simulink model "manipulator_cl"  (R2018b)
settings: Solver=ode45  StartTime=0.0  StopTime=4  RelTol=1e-6
values from neighbouring files (symbols this model uses):
  alpha_rel = 60*pi/180    (= 1.0471975512)    [parameters.m]
  kp1 = 160    [parameters.m]
  kp2 = 60    [parameters.m]
  kv1 = 11    [parameters.m]
  kv2 = 1.1    [parameters.m]
  rad_deg = 180/pi    (= 57.2957795131)    [parameters.m]
  sys_titop = directDynamicsSuper*tf(1, [1 0])    [titop_model.m]
undefined symbols (not defined in the file or in its folder): sys_phode
settings Model: Creator=a.brugnoli  LastModifiedBy=a.brugnoli

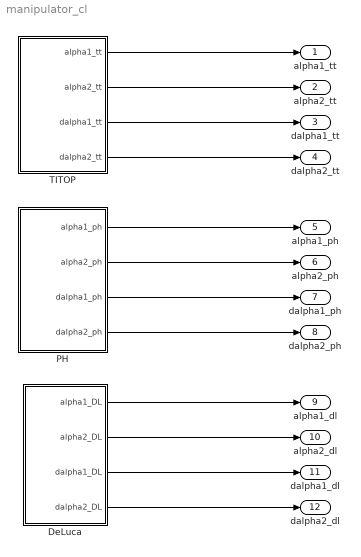
== system manipulator_cl ==
  DeLuca : Subsystem
  PH : Subsystem
  TITOP : Subsystem
  alpha1_tt : Outport
  alpha2_tt : Outport  Port=2
  dalpha1_tt : Outport  Port=3
  dalpha2_tt : Outport  Port=4
  alpha1_ph : Outport  Port=5
  alpha2_ph : Outport  Port=6
  dalpha1_ph : Outport  Port=7
  dalpha2_ph : Outport  Port=8
  alpha1_dl : Outport  Port=9
  alpha2_dl : Outport  Port=10
  dalpha1_dl : Outport  Port=11
  dalpha2_dl : Outport  Port=12
  wires:
  TITOP/1(alpha1_tt) -> alpha1_tt/1
  TITOP/2(alpha2_tt) -> alpha2_tt/1
  TITOP/3(dalpha1_tt) -> dalpha1_tt/1
  TITOP/4(dalpha2_tt) -> dalpha2_tt/1
  PH/1(alpha1_ph) -> alpha1_ph/1
  PH/2(alpha2_ph) -> alpha2_ph/1
  PH/3(dalpha1_ph) -> dalpha1_ph/1
  PH/4(dalpha2_ph) -> dalpha2_ph/1
  DeLuca/1(alpha1_DL) -> alpha1_dl/1
  DeLuca/2(alpha2_DL) -> alpha2_dl/1
  DeLuca/3(dalpha1_DL) -> dalpha1_dl/1
  DeLuca/4(dalpha2_DL) -> dalpha2_dl/1

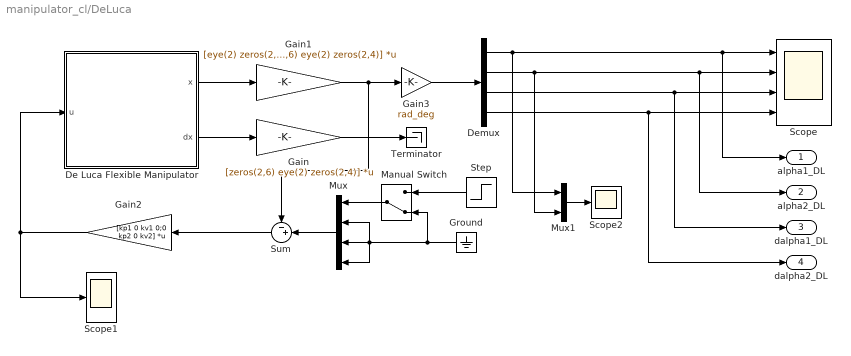
== system manipulator_cl/DeLuca ==
  De Luca Flexible Manipulator : Subsystem
  Demux : Demux
  Gain : Gain  Gain=[zeros(2,6) eye(2) zeros(2,4)]  Multiplication=Matrix(K*u) (u vector)
  Gain1 : Gain  Gain=[eye(2) zeros(2,10); zeros(2,6) eye(2) zeros(2,4)]  Multiplication=Matrix(K*u) (u vector)
  Gain2 : Gain  Gain="[kp1 0 kv1 0;0  kp2 0  kv2]"  Multiplication=Matrix(K*u) (u vector)
  Gain3 : Gain  Gain=rad_deg
  Ground : Ground
  Manual Switch : ManualSwitch  CurrentSetting=0
  Mux : Mux
  Mux1 : Mux  Inputs=2
  Scope : Scope  NumInputPorts=4
  Scope1 : Scope
  Scope2 : Scope
  Step : Step  After=alpha_rel  SampleTime=0
  Sum : Sum  Inputs=-+|
  Terminator : Terminator
  alpha1_DL : Outport
  alpha2_DL : Outport  Port=2
  dalpha1_DL : Outport  Port=3
  dalpha2_DL : Outport  Port=4
  wires:
  Gain/1 -> Terminator/1
  Mux1/1 -> Scope2/1
  Step/1 -> Manual Switch/1
  De Luca Flexible Manipulator/2(dx) -> Gain/1
  Mux/1 -> Sum/2
  Demux/1 -> alpha1_DL/1, Scope/1, Mux1/1
  Gain2/1 -> Scope1/1, De Luca Flexible Manipulator/1(u)
  Demux/2 -> alpha2_DL/1, Scope/2, Mux1/2
  Gain1/1 -> Gain3/1, Sum/1
  Demux/3 -> dalpha1_DL/1, Scope/3
  De Luca Flexible Manipulator/1(x) -> Gain1/1
  Gain3/1 -> Demux/1
  Ground/1 -> Manual Switch/2, Mux/2, Mux/4, Mux/3
  Demux/4 -> dalpha2_DL/1, Scope/4
  Sum/1 -> Gain2/1
  Manual Switch/1 -> Mux/1

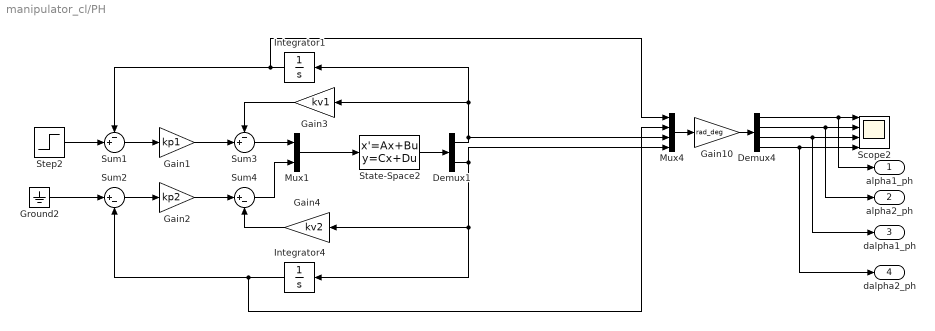
== system manipulator_cl/PH ==
  Demux1 : Demux  Outputs=2
  Demux4 : Demux
  Gain1 : Gain  Gain=kp1
  Gain10 : Gain  Gain=rad_deg
  Gain2 : Gain  Gain=kp2
  Gain3 : Gain  Gain=kv1
  Gain4 : Gain  Gain=kv2
  Ground2 : Ground
  Integrator1 : Integrator
  Integrator4 : Integrator
  Mux1 : Mux  Inputs=2
  Mux4 : Mux
  Scope2 : Scope  NumInputPorts=4
  State-Space2 : StateSpace  A=sys_phode.A  B=sys_phode.B  C=sys_phode.C  D=sys_phode.D  InitialCondition=0
  Step2 : Step  After=alpha_rel  SampleTime=0
  Sum1 : Sum  Inputs=-+|
  Sum2 : Sum  Inputs=|+-
  Sum3 : Sum  Inputs=-+|
  Sum4 : Sum  Inputs=|+-
  alpha1_ph : Outport
  alpha2_ph : Outport  Port=2
  dalpha1_ph : Outport  Port=3
  dalpha2_ph : Outport  Port=4
  wires:
  Gain1/1 -> Sum3/2
  Mux4/1 -> Gain10/1
  Gain3/1 -> Sum3/1
  Gain2/1 -> Sum4/1
  Demux4/1 -> alpha1_ph/1, Scope2/1
  Gain10/1 -> Demux4/1
  Sum2/1 -> Gain2/1
  Ground2/1 -> Sum2/1
  Sum1/1 -> Gain1/1
  Demux4/4 -> dalpha2_ph/1, Scope2/4
  Demux1/2 -> Integrator4/1, Gain4/1, Mux4/4
  Demux4/2 -> alpha2_ph/1, Scope2/2
  Integrator1/1 -> Mux4/1, Sum1/1
  Integrator4/1 -> Mux4/2, Sum2/2
  Step2/1 -> Sum1/2
  Demux1/1 -> Gain3/1, Integrator1/1, Mux4/3
  Mux1/1 -> State-Space2/1
  Demux4/3 -> dalpha1_ph/1, Scope2/3
  Sum4/1 -> Mux1/2
  Sum3/1 -> Mux1/1
  State-Space2/1 -> Demux1/1
  Gain4/1 -> Sum4/2

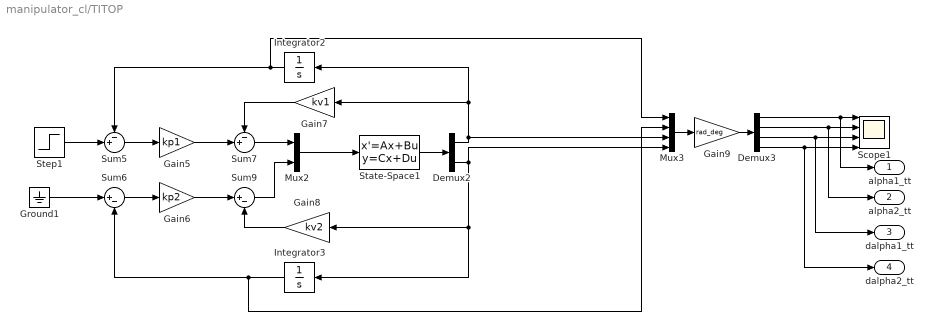
== system manipulator_cl/TITOP ==
  Demux2 : Demux  Outputs=2
  Demux3 : Demux
  Gain5 : Gain  Gain=kp1
  Gain6 : Gain  Gain=kp2
  Gain7 : Gain  Gain=kv1
  Gain8 : Gain  Gain=kv2
  Gain9 : Gain  Gain=rad_deg
  Ground1 : Ground
  Integrator2 : Integrator
  Integrator3 : Integrator
  Mux2 : Mux  Inputs=2
  Mux3 : Mux
  Scope1 : Scope  NumInputPorts=4
  State-Space1 : StateSpace  A=sys_titop.A  B=sys_titop.B  C=sys_titop.C  D=sys_titop.D  InitialCondition=0
  Step1 : Step  After=alpha_rel  SampleTime=0
  Sum5 : Sum  Inputs=-+|
  Sum6 : Sum  Inputs=|+-
  Sum7 : Sum  Inputs=-+|
  Sum9 : Sum  Inputs=|+-
  alpha1_tt : Outport
  alpha2_tt : Outport  Port=2
  dalpha1_tt : Outport  Port=3
  dalpha2_tt : Outport  Port=4
  wires:
  Gain5/1 -> Sum7/2
  Ground1/1 -> Sum6/1
  Gain7/1 -> Sum7/1
  State-Space1/1 -> Demux2/1
  Gain8/1 -> Sum9/2
  Demux3/3 -> dalpha1_tt/1, Scope1/3
  Demux2/1 -> Gain7/1, Integrator2/1, Mux3/3
  Integrator3/1 -> Mux3/2, Sum6/2
  Integrator2/1 -> Mux3/1, Sum5/1
  Sum9/1 -> Mux2/2
  Gain9/1 -> Demux3/1
  Demux2/2 -> Integrator3/1, Gain8/1, Mux3/4
  Demux3/4 -> dalpha2_tt/1, Scope1/4
  Mux3/1 -> Gain9/1
  Sum5/1 -> Gain5/1
  Sum7/1 -> Mux2/1
  Demux3/2 -> alpha2_tt/1, Scope1/2
  Mux2/1 -> State-Space1/1
  Sum6/1 -> Gain6/1
  Demux3/1 -> alpha1_tt/1, Scope1/1
  Gain6/1 -> Sum9/1
  Step1/1 -> Sum5/2

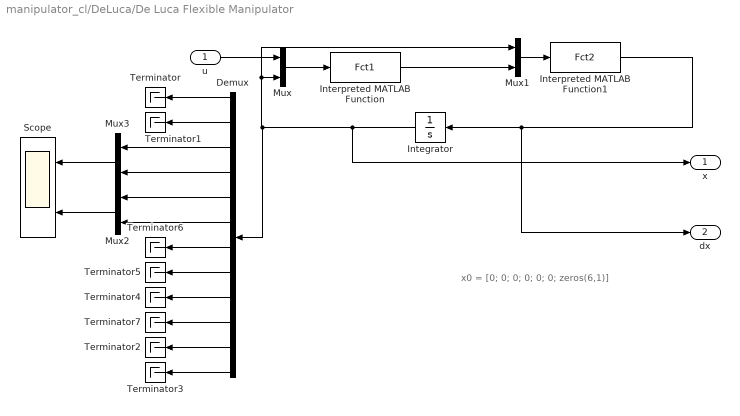
== system manipulator_cl/DeLuca/De Luca Flexible Manipulator ==
  note: x0 = [0; 0; 0; 0; 0; 0; zeros(6,1)]
  u : Inport  PortDimensions=2
  Demux : Demux  Outputs=12
  Integrator : Integrator  InitialCondition="[0; 0; 0; 0; 0; 0;  zeros(6,1);]"
  Interpreted MATLAB Function : MATLABFcn  MATLABFcn=Fct1  OutputDimensions=12
  Interpreted MATLAB Function1 : MATLABFcn  MATLABFcn=Fct2  OutputDimensions=12
  Mux : Mux  Inputs=[2 12]
  Mux1 : Mux  Inputs=[12 12]
  Mux2 : Mux  Inputs=2
  Mux3 : Mux  Inputs=2
  Scope : Scope  NumInputPorts=2
  Terminator{,1..7} (8 alike) : Terminator
  x : Outport  PortDimensions=12
  dx : Outport  Port=2  PortDimensions=12
  wires:
  u/1 -> Mux/1
  Interpreted MATLAB Function1/1 -> dx/1, Integrator/1
  Mux/1 -> Interpreted MATLAB Function/1
  Interpreted MATLAB Function/1 -> Mux1/2
  Integrator/1 -> x/1, Demux/1, Mux1/1, Mux/2
  Mux1/1 -> Interpreted MATLAB Function1/1
  Demux/3 -> Mux3/1
  Demux/4 -> Mux3/2
  Demux/5 -> Mux2/1
  Demux/6 -> Mux2/2
  Mux3/1 -> Scope/1
  Mux2/1 -> Scope/2
  Demux/1 -> Terminator/1
  Demux/2 -> Terminator1/1
  Demux/7 -> Terminator6/1
  Demux/8 -> Terminator5/1
  Demux/9 -> Terminator4/1
  Demux/10 -> Terminator7/1
  Demux/11 -> Terminator2/1
  Demux/12 -> Terminator3/1
